simulink model "sampleModel310"  (R2021b)
settings: Solver=VariableStepAuto  StartTime=0.0  StopTime=10.0  RelTol=1e-3
undefined symbols (not defined in the file or in its folder): Newton, Raphson
libraries: simulink x3, slpidlib x1
settings Model: Creator=user  LastModifiedBy=user

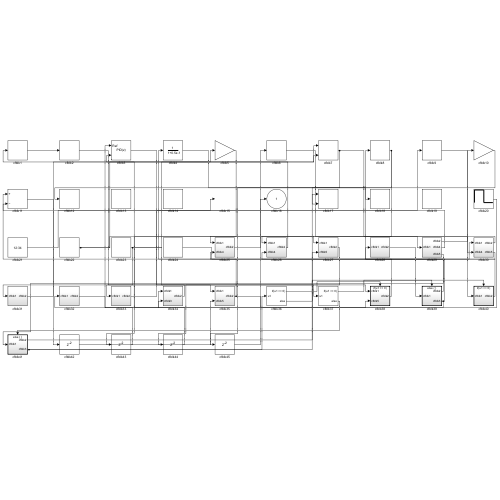
[thumbnail: Simulink's stored preview of the top-level diagram]
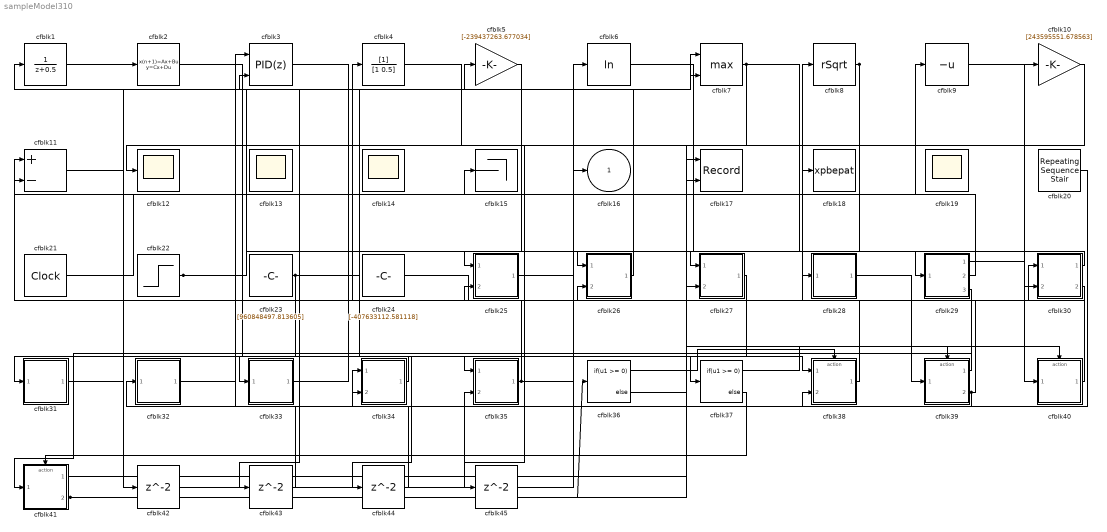
== system sampleModel310 ==
  cfblk1 : DiscreteTransferFcn  SampleTime=1
  cfblk10 : Gain  Gain=[243595551.678563]
  cfblk11 : Sum  Inputs=+-
  cfblk{12..14,19} (4 alike) : Scope
      cfblk13 settings: Floating=on
      cfblk14 settings: Floating=on
      cfblk19 settings: Floating=on
  cfblk15 : Terminator
  cfblk17 : Record  FileSettingsInternal="{\"entries\":[{\"content\":{\"excelSettings\":{\"content\":{},\"type\":\"Streamout.ExcelSettings\"}},\"type\":\"Streamout.FileSettingStorage\",\"uuid\":\"312a10b1-89cf-4c5c-a621-01bc6cabde5f\"}],\"packageUris\":[\"http://schema.mathworks.com/mf0/streamout_blocks/R2020a\"],\"version\":\"1.0\"}"  Layout=[1 1]  SignalsInternal="{\"entries\":[{\"content\":{\"signals\":[{\"content\":{\"blockPath\":[\"sampleModel310/cfblk17\"],\"channel\":[],\"dimensions\":[1],\"domain\":\"sampleModel310/cfblk17\",\"lineColor\":\"#a2142f\",\"plots\":[1],\"port\":1,\"sid\":[\"\"],\"signalID\":13147,\"signalName\":\"cfblk41:1\"},\"type\":\"RecordBlkView.Signal\",\"uuid\":\"c7fc858c-845e-4c1e-8d54-91662f97e470\"},{\"content\":{\"blockPath\":[\"sampleModel310/cfblk17\"],\"channel\":[],\"dimensions\":[1],\"domain\":\"sampleModel310/cfblk17\",\"lineColor\":\"#139fff\",\"plots\":[1],\"port\":2,\"sid\":[\"\"],\"signalID\":13151,\"signalName\":\"cfblk7\"},\"type\":\"RecordBlkView.Signal\",\"uuid\":\"02c37114-f0a3-40b2-89f3-01bf2ee586af\"}]},\"type\":\"RecordBlkView.InputSignals\",\"uuid\":\"c0784377-5317-4dc0-a00d-cdafa8f4d3c4\"}],\"packageUris\":[\"http://schema.mathworks.com/mf0/streamout_blocks/R2020a\"],\"version\":\"1.0\"}"  VisualizationBindings="{\"xyplotplugin\":{\"info\":[{\"series\":[{\"bindingParametersList\":[{\"parameter\":\"X-Axis\",\"signalID\":13147,\"signalName\":\"cfblk41:1\"},{\"parameter\":\"Y-Axis\",\"signalID\":13151,\"signalName\":\"cfblk7\"}],\"seriesID\":13952}],\"subplotID\":1}]}}"  CompatibilityTag=XY
  cfblk18 : ToWorkspace  VariableName=xpbepat  SaveFormat=Timeseries  SampleTime=-1
  cfblk2 : DiscreteStateSpace
  cfblk20 : simulink/Sources/Repeating Sequence Stair  OutValues=[-260257791.293506, -984916675.448606]  tsamp=-1  OutMin=[]  OutMax=[]  OutDataTypeStr=double  OutputDataTypeScalingMode=double  OutDataType=fixdt(0,8)  ConRadixGroup=Best Precision: Vector-wise  OutScaling=2^-12
  cfblk21 : DigitalClock
  cfblk22 : Step  Time=[35.000000]  Before=[-147491021.579272]  After=[-949046595.785974]  SampleTime=0
  cfblk23 : Constant  Value=[960848497.813605]  SampleTime=1
  cfblk24 : Constant  Value=[-407633112.581118]  SampleTime=1
  cfblk25 : Subsystem
  cfblk26 : Subsystem
  cfblk27 : Subsystem
  cfblk28 : Subsystem
  cfblk29 : Subsystem
  cfblk3 : slpidlib/PID Controller (2DOF)  Controller=PID  Form=Parallel  TimeDomain=Discrete-time  UseExternalTs=off  SampleTime=1  IntegratorMethod=Forward Euler  FilterMethod=Forward Euler  ControllerParametersSource=internal  P=1  I=1  D=0  UseFilter=on  N=100  b=1  c=1  TunerSelectOption=Transfer Function Based (PID Tuner App)  InitialConditionSource=internal  InitialConditionForIntegrator=0  InitialConditionForFilter=0  DifferentiatorICPrevScaledInput=0  ExternalReset=none  TrackingMode=off  Kt=1  LimitOutput=off  SatLimitsSource=internal  UpperSaturationLimit=inf  LowerSaturationLimit=-inf  LinearizeAsGain=off  AntiWindupMode=none  Kb=1  POutMin=[]  POutMax=[]  IOutMin=[]  IOutMax=[]  DOutMin=[]  DOutMax=[]  NOutMin=[]  NOutMax=[]  bOutMin=[]  bOutMax=[]  cOutMin=[]  cOutMax=[]  SumOutMin=[]  SumOutMax=[]  SaturationOutMin=[]  SaturationOutMax=[]  PParamMin=[]  PParamMax=[]  IParamMin=[]  IParamMax=[]  DParamMin=[]  DParamMax=[]  NParamMin=[]  NParamMax=[]  bParamMin=[]  bParamMax=[]  cParamMin=[]  cParamMax=[]  KbParamMin=[]  KbParamMax=[]  KtParamMin=[]  KtParamMax=[]  KbOutMin=[]  KbOutMax=[]  KtOutMin=[]  KtOutMax=[]  IntegratorOutMin=[]  IntegratorOutMax=[]  FilterOutMin=[]  FilterOutMax=[]  SumI1OutMin=[]  SumI1OutMax=[]  SumI2OutMin=[]  SumI2OutMax=[]  SumI3OutMin=[]  SumI3OutMax=[]  SumI4OutMin=[]  SumI4OutMax=[]  SumDOutMin=[]  SumDOutMax=[]  Sum1OutMin=[]  Sum1OutMax=[]  Sum2OutMin=[]  Sum2OutMax=[]  Sum3OutMin=[]  Sum3OutMax=[]  DifferentiatorOutMin=[]  DifferentiatorOutMax=[]  FilterDiffOutCoefMin=[]  FilterDiffOutCoefMax=[]  ReciprocalOutMin=[]  ReciprocalOutMax=[]  SumDenOutMin=[]  SumDenOutMax=[]  SumNumOutMin=[]  SumNumOutMax=[]  DivideOutMin=[]  DivideOutMax=[]  UdiffTsProdOutMin=[]  UdiffTsProdOutMax=[]  NTsProdOutMin=[]  NTsProdOutMax=[]  UintegralTsProdOutMin=[]  UintegralTsProdOutMax=[]  UngainTsProdOutMin=[]  UngainTsProdOutMax=[]  IntegratorContinuousStateAttributes=''  IntegratorStateMustResolveToSignalObject=off  IntegratorRTWStateStorageClass=Auto  FilterContinuousStateAttributes=''  FilterStateMustResolveToSignalObject=off  FilterRTWStateStorageClass=Auto  ParallelPVariant=InternalParameters  IdealPVariant=Disabled  IVariant=InternalParameters  DVariant=InternalParameters  bVariant=InternalParameters  cVariant=InternalParameters  IntegratorVariant=Discrete  SatVariant=Disabled  AWVariant=Passthrough  PCopyVariant=Disabled  TRVariant=Disabled  FdbkBlocksVariant=Forward  IdealPFdbkVariant=Disabled  SatFdbkVariant=Disabled  DerivativeFilterVariant=ForwardEulerFilter  NVariant=InternalParameters  NCopyVariant=Disabled  FilterICVariant=InternalICsFilter  IntegratorICVariant=InternalICs  ExternalResetVariant=Disabled  TRSumVariant=Passthrough  SumFdbkVariant=Disabled  SumVariant=Sum_PID  TsampFilterVariant=InternalTs  TsampNgainVariant=Passthrough  TsampIntegralVariant=Passthrough  ExternalSaturationOutDataTypeStr=Inherit: Same as second input
      settings: SourceProductBaseCode=SL
  cfblk30 : Subsystem
  cfblk31 : Subsystem
  cfblk32 : Subsystem
  cfblk33 : Subsystem
  cfblk34 : Subsystem
  cfblk35 : Subsystem
  cfblk36 : If  IfExpression=u1 >= 0  SampleTime=1
  cfblk37 : If  IfExpression=u1 >= 0  SampleTime=1
  cfblk38 : Subsystem  TreatAsAtomicUnit=on
  cfblk39 : Subsystem  TreatAsAtomicUnit=on
  cfblk4 : DiscreteFilter  SampleTime=1
  cfblk40 : Subsystem  TreatAsAtomicUnit=on
  cfblk41 : Subsystem  TreatAsAtomicUnit=on
  cfblk{42..45} (4 alike) : Delay  SampleTime=1
  cfblk5 : Gain  Gain=[-239437263.677034]
  cfblk6 : Math  Operator=log  SaturateOnIntegerOverflow=on
  cfblk7 : MinMax  Function=max  Inputs=2
  cfblk8 : Sqrt  Operator=rSqrt  AlgorithmType=Newton-Raphson  SaturateOnIntegerOverflow=on
  cfblk9 : UnaryMinus
  cfblk16 : Outport
  wires:
  cfblk26/1(cfblk2) -> cfblk1/1
  cfblk2/1 -> cfblk35/1(cfblk1)
  cfblk24/1 -> cfblk30/1(cfblk1)
  cfblk21/1 -> cfblk9/1
  cfblk20/1 -> cfblk32/1(cfblk1)
  cfblk35/1(cfblk2) -> cfblk4/1, cfblk38/2(cfblk5)
  cfblk39/1(cfblk2) -> cfblk8/1
  cfblk30/1(cfblk2) -> cfblk25/1(cfblk1)
  cfblk39/2(cfblk3) -> cfblk34/1(cfblk1), cfblk26/2(cfblk4)
  cfblk33/1(cfblk2) -> cfblk15/1
  cfblk3/1 -> cfblk37/1
  cfblk30/2(cfblk5) -> cfblk28/1(cfblk1)
  cfblk23/1 -> cfblk33/1(cfblk1), cfblk38/1(cfblk1), cfblk7/2
  cfblk34/1(cfblk2) -> cfblk31/1(cfblk1)
  cfblk9/1 -> cfblk40/1(cfblk1)
  cfblk40/1(cfblk2) -> cfblk25/2(cfblk4)
  cfblk29/1(cfblk2) -> cfblk10/1
  cfblk1/1 -> cfblk2/1
  cfblk22/1 -> cfblk27/1(cfblk1), cfblk7/1
  cfblk7/1 -> cfblk30/2(cfblk4), cfblk17/2
  cfblk31/1(cfblk2) -> cfblk5/1
  cfblk6/1 -> cfblk29/1(cfblk1)
  cfblk4/1 -> cfblk18/1
  cfblk8/1 -> cfblk26/1(cfblk1), cfblk12/1
  cfblk32/1(cfblk2) -> cfblk34/2(cfblk3)
  cfblk25/1(cfblk2) -> cfblk16/1
  cfblk38/1(cfblk2) -> cfblk11/1
  cfblk28/1(cfblk2) -> cfblk39/1(cfblk1)
  cfblk29/2(cfblk4) -> cfblk11/2
  cfblk41/1(cfblk2) -> cfblk17/1
  cfblk29/3(cfblk5) -> cfblk41/1(cfblk1)
  cfblk41/2(cfblk3) -> cfblk36/1, cfblk27/2(cfblk5)
  cfblk36/1 -> cfblk38/Action
  cfblk36/2 -> cfblk39/Action
  cfblk37/1 -> cfblk40/Action
  cfblk37/2 -> cfblk41/Action
  cfblk11/1 -> cfblk42/1
  cfblk42/1 -> cfblk35/2(cfblk5)
  cfblk5/1 -> cfblk43/1
  cfblk43/1 -> cfblk3/1
  cfblk27/1(cfblk2) -> cfblk44/1
  cfblk44/1 -> cfblk3/2
  cfblk10/1 -> cfblk45/1
  cfblk45/1 -> cfblk6/1

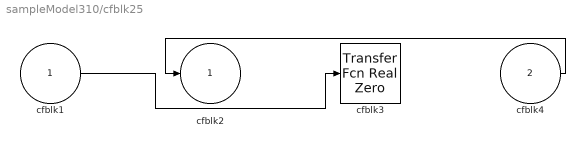
== system sampleModel310/cfblk25 ==
  cfblk1 : Inport
  cfblk4 : Inport  Port=2
  cfblk3 : simulink/Discrete/Transfer Fcn Real Zero  ZeroZ=0.75  ICPrevInput=0.0  DoSatur=off
      settings: SourceProductBaseCode=SL
  cfblk2 : Outport
  wires:
  cfblk4/1 -> cfblk2/1
  cfblk1/1 -> cfblk3/1

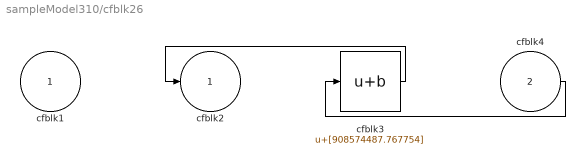
== system sampleModel310/cfblk26 ==
  cfblk1 : Inport
  cfblk4 : Inport  Port=2
  cfblk3 : Bias  Bias=[908574487.767754]
  cfblk2 : Outport
  wires:
  cfblk3/1 -> cfblk2/1
  cfblk4/1 -> cfblk3/1

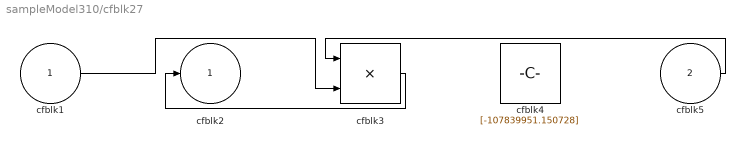
== system sampleModel310/cfblk27 ==
  cfblk1 : Inport
  cfblk5 : Inport  Port=2
  cfblk3 : Product
  cfblk4 : Constant  Value=[-107839951.150728]  SampleTime=1
  cfblk2 : Outport
  wires:
  cfblk5/1 -> cfblk3/1
  cfblk3/1 -> cfblk2/1
  cfblk1/1 -> cfblk3/2

== system sampleModel310/cfblk28 ==
  cfblk1 : Inport
  cfblk3 : Gain  Gain=[200667207.990055]
  cfblk2 : Outport
  wires:
  cfblk1/1 -> cfblk3/1
  cfblk3/1 -> cfblk2/1

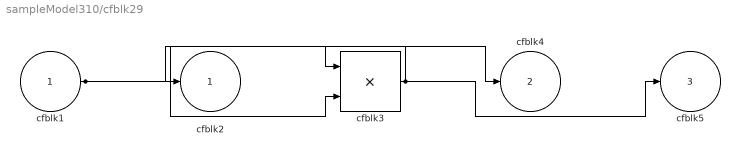
== system sampleModel310/cfblk29 ==
  cfblk1 : Inport
  cfblk3 : Product
  cfblk2 : Outport
  cfblk4 : Outport  Port=2
  cfblk5 : Outport  Port=3
  wires:
  cfblk1/1 -> cfblk4/1, cfblk3/1, cfblk3/2
  cfblk3/1 -> cfblk5/1, cfblk2/1

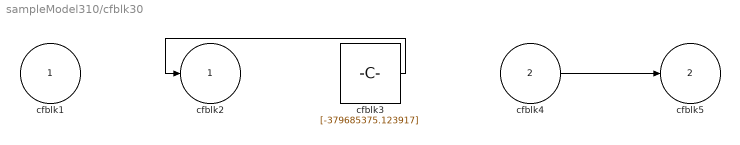
== system sampleModel310/cfblk30 ==
  cfblk1 : Inport
  cfblk4 : Inport  Port=2
  cfblk3 : Constant  Value=[-379685375.123917]  SampleTime=1
  cfblk2 : Outport
  cfblk5 : Outport  Port=2
  wires:
  cfblk3/1 -> cfblk2/1
  cfblk4/1 -> cfblk5/1

== system sampleModel310/cfblk31 ==
  cfblk1 : Inport
  cfblk3 : simulink/Discrete/Tapped Delay  vinit=0.0  samptime=-1  NumDelays=1  DelayOrder=Oldest  includeCurrent=off
  cfblk2 : Outport
  wires:
  cfblk3/1 -> cfblk2/1
  cfblk1/1 -> cfblk3/1

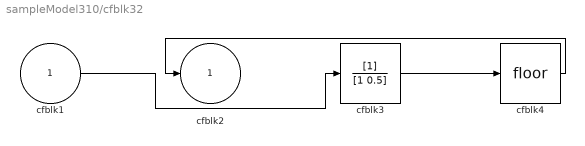
== system sampleModel310/cfblk32 ==
  cfblk1 : Inport
  cfblk3 : DiscreteFilter  SampleTime=1
  cfblk4 : Rounding
  cfblk2 : Outport
  wires:
  cfblk4/1 -> cfblk2/1
  cfblk1/1 -> cfblk3/1
  cfblk3/1 -> cfblk4/1

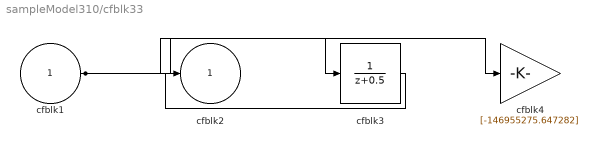
== system sampleModel310/cfblk33 ==
  cfblk1 : Inport
  cfblk3 : DiscreteTransferFcn  SampleTime=1
  cfblk4 : Gain  Gain=[-146955275.647282]
  cfblk2 : Outport
  wires:
  cfblk1/1 -> cfblk3/1, cfblk4/1
  cfblk3/1 -> cfblk2/1

== system sampleModel310/cfblk34 ==
  cfblk1 : Inport
  cfblk3 : Inport  Port=2
  cfblk2 : Outport
  wires:
  cfblk3/1 -> cfblk2/1

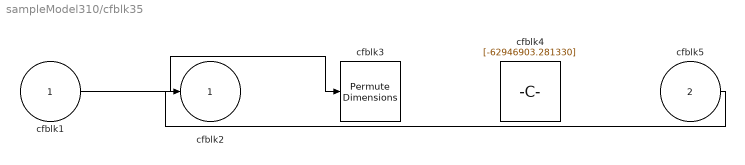
== system sampleModel310/cfblk35 ==
  cfblk1 : Inport
  cfblk5 : Inport  Port=2
  cfblk3 : PermuteDimensions
  cfblk4 : Constant  Value=[-62946903.281330]  SampleTime=1
  cfblk2 : Outport
  wires:
  cfblk1/1 -> cfblk3/1
  cfblk5/1 -> cfblk2/1

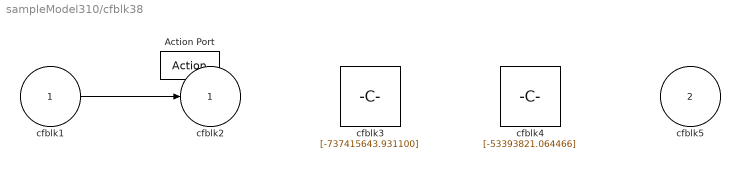
== system sampleModel310/cfblk38 ==
  cfblk1 : Inport
  cfblk5 : Inport  Port=2
  Action Port : ActionPort  ActionPortLabel=if(u1 >= 0)
  cfblk3 : Constant  Value=[-737415643.931100]  SampleTime=1
  cfblk4 : Constant  Value=[-53393821.064466]  SampleTime=1
  cfblk2 : Outport
  wires:
  cfblk1/1 -> cfblk2/1

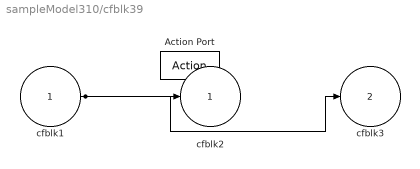
== system sampleModel310/cfblk39 ==
  cfblk1 : Inport
  Action Port : ActionPort  ActionPortLabel=else
  cfblk2 : Outport
  cfblk3 : Outport  Port=2
  wires:
  cfblk1/1 -> cfblk3/1, cfblk2/1

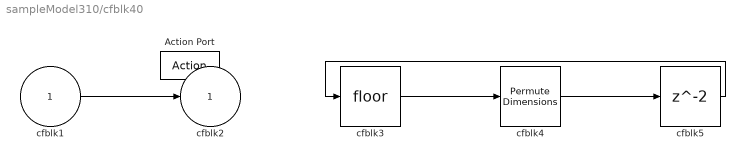
== system sampleModel310/cfblk40 ==
  cfblk1 : Inport
  Action Port : ActionPort  ActionPortLabel=if(u1 >= 0)
  cfblk3 : Rounding
  cfblk4 : PermuteDimensions
  cfblk5 : Delay
  cfblk2 : Outport
  wires:
  cfblk3/1 -> cfblk4/1
  cfblk1/1 -> cfblk2/1
  cfblk4/1 -> cfblk5/1
  cfblk5/1 -> cfblk3/1

== system sampleModel310/cfblk41 ==
  cfblk1 : Inport
  Action Port : ActionPort  ActionPortLabel=else
  cfblk2 : Outport
  cfblk3 : Outport  Port=2
  wires:
  cfblk1/1 -> cfblk2/1, cfblk3/1
